simulink model "magballdemo"  (Simulink 6.0)
settings: Solver=ode45  StartTime=0.0  StopTime=10  RelTol=1e-3
PreLoadFcn:
  | magballdat
undefined symbols (not defined in the file or in its folder): beta, L, m, R
settings Model: Creator=lparsons  LastModifiedBy=jglass  BufferReuse=off
settings DataIOCC: InitialState=x0  SignalLoggingName=logsOut
settings OptimizationCC: BlockReduction=off  InlineParams=on  BufferReuse=off
settings DebuggingCC: CheckExecutionContextPreStartOutputMsg=on  CheckExecutionContextRuntimeOutputMsg=on  SolverPrmCheckMsg=none
settings HardwareCC: TargetUnknown=on

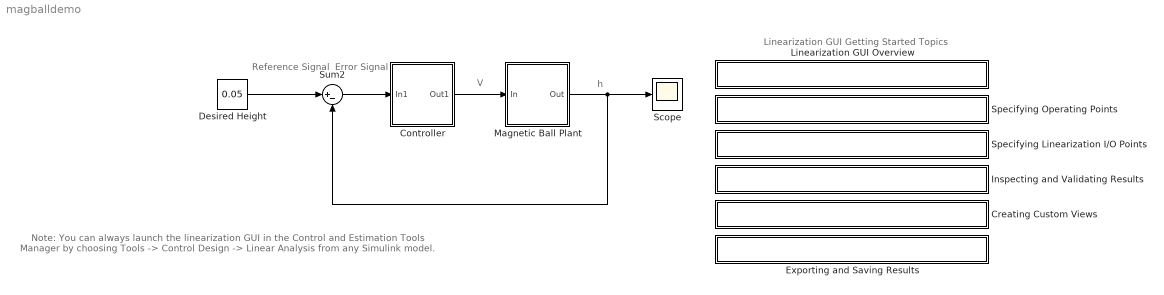
== system magballdemo ==
  note: Error
      | Signal
  note: Reference
      | Signal
  note: V
  note: h
  note: Linearization GUI Getting Started Topics
  note: Note: You can always launch the linearization GUI in the Control and Estimation Tools Manager
      | by choosing Tools -> Control Design -> Linear Analysis from any Simulink model.
  Controller : Subsystem  PropExecContextAcrossSSBoundary=on
  Creating Custom Views : Subsystem  Priority=2  PropExecContextAcrossSSBoundary=on
      settings: OpenFcn=helpview([docroot '/toolbox/slcontrol/slcontrol.map'], 'custom_views')
      mask Display: disp('Creating Custom Views')
  Desired Height : Constant  Value=0.05
  Exporting and Saving Results : Subsystem  Priority=2  PropExecContextAcrossSSBoundary=on
      settings: OpenFcn=helpview([docroot '/toolbox/slcontrol/slcontrol.map'], 'exporting')
      mask Display: disp('Exporting and Saving Results')
  Inspecting and Validating Results : Subsystem  Priority=2  PropExecContextAcrossSSBoundary=on
      settings: OpenFcn=helpview([docroot '/toolbox/slcontrol/slcontrol.map'], 'analyzing')
      mask Display: disp('Inspecting and Validating Results')
  Linearization GUI Overview : Subsystem  Priority=2  PropExecContextAcrossSSBoundary=on
      settings: OpenFcn=helpview([docroot '/toolbox/slcontrol/slcontrol.map'], 'linearizing_models')
      mask Display: disp('Linearization GUI Overview')
  Magnetic Ball Plant : Subsystem  PropExecContextAcrossSSBoundary=on
  Scope : Scope
  Specifying Linearization I/O Points : Subsystem  Priority=2  PropExecContextAcrossSSBoundary=on
      settings: OpenFcn=helpview([docroot '/toolbox/slcontrol/slcontrol.map'], 'analysis_ios')
      mask Display: disp('Specifying Linearization I/O Points')
  Specifying Operating Points : Subsystem  Priority=2  PropExecContextAcrossSSBoundary=on
      settings: OpenFcn=helpview([docroot '/toolbox/slcontrol/slcontrol.map'], 'op_points')
      mask Display: disp('Specifying Operating Points')
  Sum2 : Sum  Inputs=|+-
  wires:
  Magnetic Ball Plant/1(Out) -> Scope/1, Sum2/2
  Sum2/1 -> Controller/1(In1)
  Controller/1(Out1) -> Magnetic Ball Plant/1(In)
  Desired Height/1 -> Sum2/1

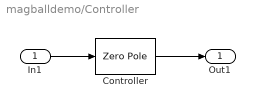
== system magballdemo/Controller ==
  In1 : Inport  LatchInput=off
  Controller : ZeroPole  Zeros=[-11.5000+5.7900i,-11.5000-5.7900i]  Poles=[0 -1000]  Gain=-3.3057e+004
  Out1 : Outport
  wires:
  In1/1 -> Controller/1
  Controller/1 -> Out1/1

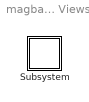
== system magballdemo/Creating Custom Views ==
  Subsystem : Subsystem  PropExecContextAcrossSSBoundary=on

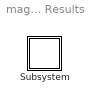
== system magballdemo/Exporting and Saving Results ==
  Subsystem : Subsystem  PropExecContextAcrossSSBoundary=on

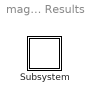
== system magballdemo/Inspecting and Validating Results ==
  Subsystem : Subsystem  PropExecContextAcrossSSBoundary=on

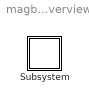
== system magballdemo/Linearization GUI Overview ==
  Subsystem : Subsystem  PropExecContextAcrossSSBoundary=on

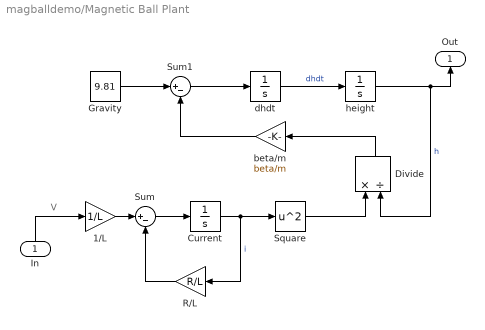
== system magballdemo/Magnetic Ball Plant ==
  note: V
  In : Inport  Orientation=up  LatchInput=off
  1/L : Gain  Gain=1/L
  Current : Integrator  InitialCondition=7.0036
  Divide : Product  Orientation=up  Inputs=*/  OutScaling=2^-10
  Gravity : Constant  Value=9.81
  R/L : Gain  Orientation=left  Gain=R/L
  Square : Math  Operator=square  SaturateOnIntegerOverflow=on
  Sum : Sum  Inputs=|+-
  Sum1 : Sum  Inputs=|+-
  beta/m : Gain  Orientation=left  Gain=beta/m
  dhdt : Integrator
  height : Integrator  InitialCondition=0.05
  Out : Outport  Orientation=up
  wires:
  dhdt/1 -> height/1  "dhdt"
  height/1 -> Out/1, Divide/2  "h"
  Sum/1 -> Current/1
  1/L/1 -> Sum/1
  R/L/1 -> Sum/2
  Current/1 -> Square/1, R/L/1  "i"
  Square/1 -> Divide/1
  Divide/1 -> beta/m/1
  Gravity/1 -> Sum1/1
  beta/m/1 -> Sum1/2
  Sum1/1 -> dhdt/1
  In/1 -> 1/L/1

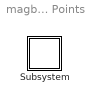
== system magballdemo/Specifying Linearization I/O Points ==
  Subsystem : Subsystem  PropExecContextAcrossSSBoundary=on

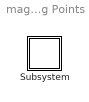
== system magballdemo/Specifying Operating Points ==
  Subsystem : Subsystem  PropExecContextAcrossSSBoundary=on

== system magballdemo/Creating Custom Views/Subsystem ==

== system magballdemo/Exporting and Saving Results/Subsystem ==

== system magballdemo/Inspecting and Validating Results/Subsystem ==

== system magballdemo/Linearization GUI Overview/Subsystem ==

== system magballdemo/Specifying Linearization I/O Points/Subsystem ==

== system magballdemo/Specifying Operating Points/Subsystem ==
